simulink model "Overforingsfunksjon_Phi_PID_med_forstyrrelse"  (R2023b)
settings: Solver=ode1  StartTime=0.0  StopTime=10  FixedStep=1/30000  RelTol=1e-8
values from neighbouring files (symbols this model uses):
  D_phi = [M(4),rho_vann*Cd*A_phi*phi_2,(Zm*G-Zb*F_b)*cosd(thetha)*cosd(phi_1)]    [Overforingsfunksjon_Rotasjon.m]
settings Model: Creator=Anne Brit  LastModifiedBy=anneb
settings DataIOCC: InitialState=0.5

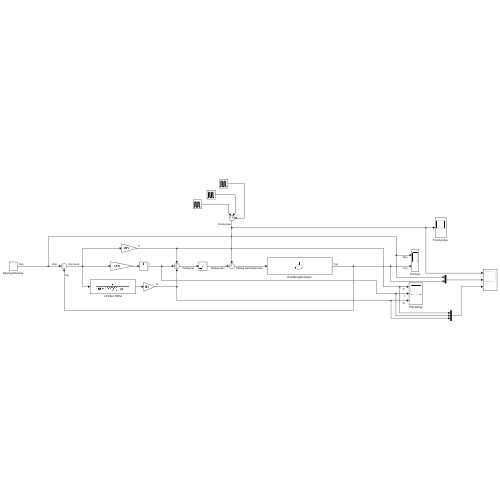
[thumbnail: Simulink's stored preview of the top-level diagram]
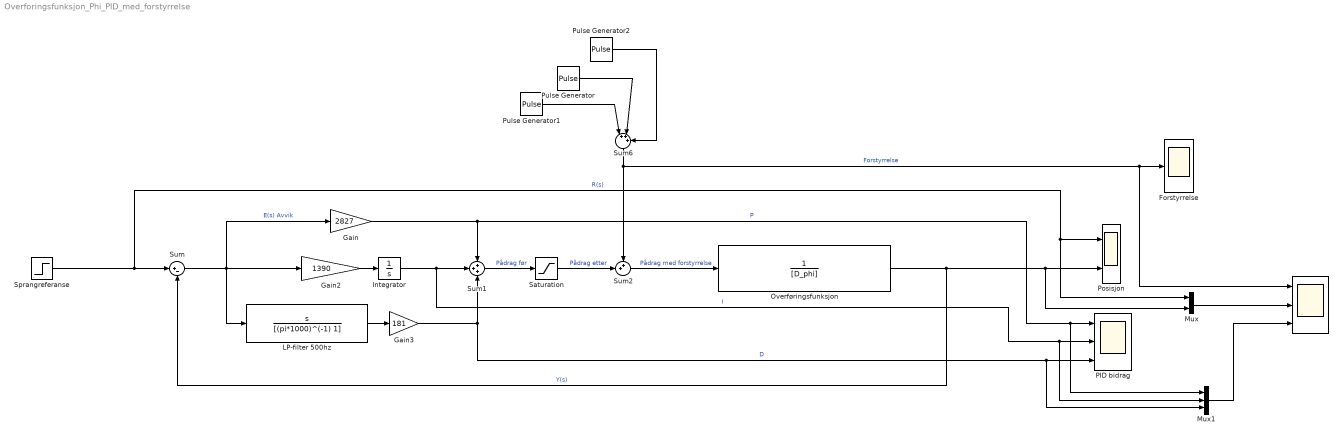
== system Overforingsfunksjon_Phi_PID_med_forstyrrelse ==
  " " : Scope  NumInputPorts=3
  " LP-filter 500hz" : TransferFcn  Numerator=[1 0]  Denominator=[(pi*1000)^(-1) 1]
  Forstyrrelse : Scope
  Gain : Gain  Gain=2827
  Gain2 : Gain  Gain=1390
  Gain3 : Gain  Gain=181
  Integrator : Integrator
  Mux : Mux  Inputs=2
  Mux1 : Mux  Inputs=3
  "Overføringsfunksjon " : TransferFcn  Denominator=[D_phi]
  PID bidrag : Scope  NumInputPorts=3
  Posisjon : Scope  NumInputPorts=2
  Pulse Generator : DiscretePulseGenerator  PulseType=Time based  Amplitude=5  Period=10  PulseWidth=5  PhaseDelay=3
  Pulse Generator1 : DiscretePulseGenerator  PulseType=Time based  Amplitude=5  Period=10  PhaseDelay=1
  Pulse Generator2 : DiscretePulseGenerator  PulseType=Time based  Amplitude=5  Period=10  PulseWidth=10  PhaseDelay=6
  Saturation : Saturate  UpperLimit=350  LowerLimit=-345
  Sprangreferanse : Step  After=0  SampleTime=0
  Sum : Sum  Inputs=|+-
  Sum1 : Sum  Inputs=+++
  Sum2 : Sum  Inputs=++|
  Sum6 : Sum  Inputs=|+++
  wires:
  "Overføringsfunksjon "/1 -> Sum/2, Mux/2, Posisjon/2  "Y(s)"
  Gain2/1 -> Integrator/1
  Sum/1 -> " LP-filter 500hz"/1, Gain/1, Gain2/1  "E(s) Avvik"
  Gain/1 -> Mux1/1, PID bidrag/1, Sum1/1  "P"
  Gain3/1 -> Sum1/3, Mux1/3, PID bidrag/3  "D"
  Sprangreferanse/1 -> Mux/1, Posisjon/1, Sum/1  "R(s)"
  Integrator/1 -> Mux1/2, PID bidrag/2, Sum1/2  "I"
  " LP-filter 500hz"/1 -> Gain3/1
  Saturation/1 -> Sum2/2  "Pådrag etter"
  Sum1/1 -> Saturation/1  "Pådrag før"
  Sum2/1 -> "Overføringsfunksjon "/1  "Pådrag med forstyrrelse"
  Pulse Generator1/1 -> Sum6/1
  Pulse Generator/1 -> Sum6/2
  Sum6/1 -> " "/1, Forstyrrelse/1, Sum2/1  "Forstyrrelse"
  Pulse Generator2/1 -> Sum6/3
  Mux/1 -> " "/2
  Mux1/1 -> " "/3
